simulink model "InverterTestCell2"  (R2021a)
settings: Solver=FixedStepAuto  StartTime=0.0  StopTime=860  FixedStep=0.005  RelTol=1e-3
values from neighbouring files (symbols this model uses):
  ACderate = 0.7910    (= 0.791)    [simvar.m]
  CoreDm = 0.07    [simvar.m]
  CoreRm = 0.250/2    (= 0.125)    [simvar.m]
  Di = 0.085    [Optomised_simvar.m]    (also in simvar.m)
  Dm = 0.08    [simvar.m]
  Hi = 0.250    (= 0.25)    [Optomised_simvar.m]    (also in simvar.m)
  La = 1    [Optomised_simvar.m]    (also in simvar.m = 1.5)
  Li = 0.488    [Optomised_simvar.m]    (also in simvar.m)
  Lw = 1    [Optomised_simvar.m]    (also in simvar.m = 1.5)
  PDi = 0.03    [Optomised_simvar.m]    (also in simvar.m = 0.01)
  PDm = 0.01    [simvar.m]
  PLi = 1    [Optomised_simvar.m]    (also in simvar.m = 3.2)
  PLm = 0.721    [simvar.m]
  PSplit = 0.95    [simvar.m]
  Rm = 0.268/2    (= 0.134)    [simvar.m]
  StartTempI = 295    [simvar.m]
  StartTempM = 291    [simvar.m]
libraries: fl_lib x45, nesl_utility x17
settings Model: PacingRate=0.001800  Creator=Henry  LastModifiedBy=Henry

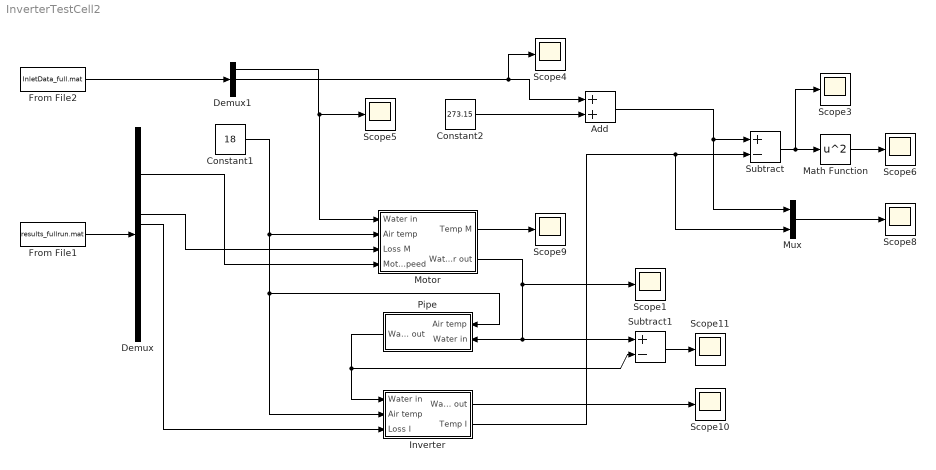
== system InverterTestCell2 ==
  Add : Sum
  Constant1 : Constant  Value=18
  Constant2 : Constant  Value=273.15
  Demux : Demux  Outputs=19
  Demux1 : Demux  Outputs=3
  From File1 : FromFile  FileName=results_fullrun.mat  SampleTime=0
  From File2 : FromFile  FileName=InletData_full.mat  SampleTime=0
  Inverter : Subsystem
  Math Function : Math  Operator=square  SaturateOnIntegerOverflow=on
  Motor : Subsystem
  Mux : Mux  Inputs=2
  Pipe : Subsystem
  Scope{1,3..6,8..11} (9 alike) : Scope
  Subtract : Sum  Inputs=+-
  Subtract1 : Sum  Inputs=+-
  wires:
  From File1/1 -> Demux/1
  Inverter/2(Temp I) -> Mux/2, Subtract/2
  Constant1/1 -> Motor/2(Air temp), Inverter/2(Air temp), Pipe/1(Air temp)
  From File2/1 -> Demux1/1
  Add/1 -> Subtract/1, Mux/1
  Constant2/1 -> Add/2
  Subtract/1 -> Math Function/1, Scope3/1
  Math Function/1 -> Scope6/1
  Mux/1 -> Scope8/1
  Motor/2(Water out) -> Subtract1/1, Pipe/2(Water in), Scope1/1
  Demux/9 -> Inverter/3(Loss I)
  Demux1/1 -> Motor/1(Water in), Scope5/1
  Demux1/2 -> Add/1, Scope4/1
  Demux/4 -> Motor/4(MotorSpeed)
  Demux/8 -> Motor/3(Loss M)
  Motor/1(Temp M) -> Scope9/1
  Inverter/1(Water out) -> Scope10/1
  Pipe/1(Water out) -> Inverter/1(Water in), Subtract1/2
  Subtract1/1 -> Scope11/1

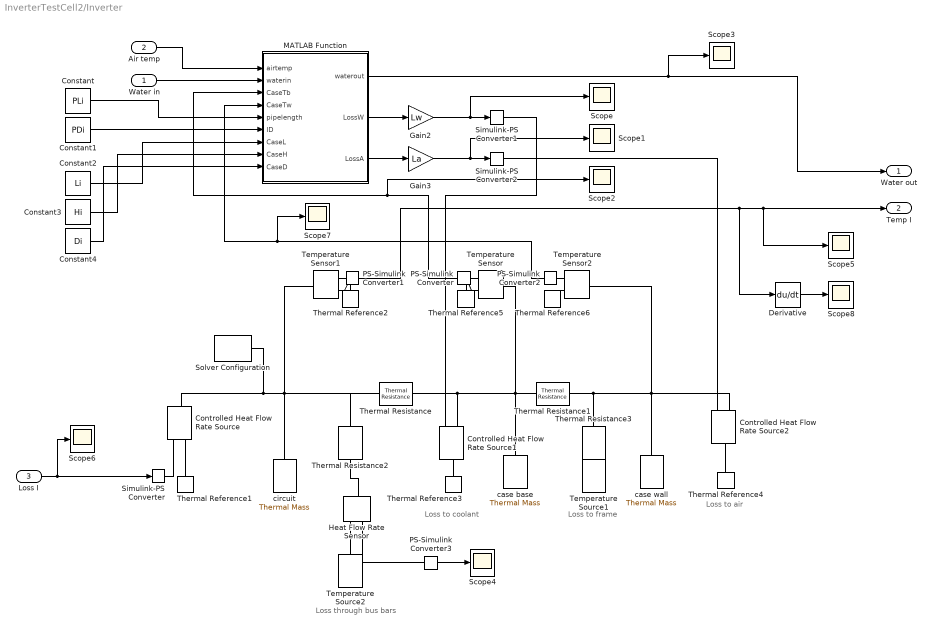
== system InverterTestCell2/Inverter ==
  note: Loss to coolant
  note: Loss to air
  note: Loss through bus
      | bars
  note: Loss to frame
  Water in : Inport
  Air temp : Inport  Port=2
  Loss I : Inport  Port=3
  " case base" : fl_lib/Thermal/Thermal Elements/Thermal Mass  mass=MIbf kg  sp_heat=CpIb J/kg/K  T_specify=on  T_priority=High  T=StartTempI K  T_nominal_specify=off  T_nominal_unit=K  T_nominal_value=1  Q_specify=off  Q_priority=None  Q=0 W  Q_nominal_specify=off  Q_nominal_unit=W  Q_nominal_value=1
  " case wall" : fl_lib/Thermal/Thermal Elements/Thermal Mass  mass=MIbw kg  sp_heat=CpIb J/kg/K  T_specify=on  T_priority=High  T=StartTempI K  T_nominal_specify=off  T_nominal_unit=K  T_nominal_value=1  Q_specify=off  Q_priority=None  Q=0 W  Q_nominal_specify=off  Q_nominal_unit=W  Q_nominal_value=1
  Constant : Constant  Value=PLi
  Constant1 : Constant  Value=PDi
  Constant2 : Constant  Value=Li
  Constant3 : Constant  Value=Hi
  Constant4 : Constant  Value=Di
  Controlled Heat Flow Rate Source : fl_lib/Thermal/Thermal Sources/Controlled Heat Flow Rate Source
  Controlled Heat Flow Rate Source1 : fl_lib/Thermal/Thermal Sources/Controlled Heat Flow Rate Source
  Controlled Heat Flow Rate Source2 : fl_lib/Thermal/Thermal Sources/Controlled Heat Flow Rate Source
  Derivative : Derivative
  Gain2 : Gain  Gain=Lw
  Gain3 : Gain  Gain=La
  Heat Flow Rate Sensor : fl_lib/Thermal/Thermal Sensors/Heat Flow Rate Sensor
      settings: SourceProductBaseCode=SS
  MATLAB Function : MATLAB Function  TreatAsAtomicUnit=on
  PS-Simulink Converter{,1..3} (4 alike) : nesl_utility/PS-Simulink Converter  PhysicalDomain=network_engine_domain  SubClassName=ps_output  LeftPortType=input  RightPortType=output  PseudoPeriodic=off  Frequencies=[]  Unit=inherit  AffineConversion=off
      settings: SourceProductBaseCode=PW,SS
  Scope{,1..8} (9 alike) : Scope
  Simulink-PS Converter : nesl_utility/Simulink-PS Converter  PhysicalDomain=network_engine_domain  SubClassName=ps_input  LeftPortType=input  RightPortType=output  PseudoPeriodic=off  Frequencies=[]  NoiseDistribution=none  NoiseParameters=[]  Unit=1  AffineConversion=off  FilteringAndDerivatives=provide  SimscapeFilterOrder=1  InputFilterTimeConstant=0.001  UdotUserProvided=0
      settings: SourceProductBaseCode=PW,SS
  Simulink-PS Converter1 : nesl_utility/Simulink-PS Converter  PhysicalDomain=network_engine_domain  SubClassName=ps_input  LeftPortType=input  RightPortType=output  PseudoPeriodic=off  Frequencies=[]  NoiseDistribution=none  NoiseParameters=[]  Unit=1  AffineConversion=off  FilteringAndDerivatives=provide  SimscapeFilterOrder=1  InputFilterTimeConstant=0.001  UdotUserProvided=0
      settings: SourceProductBaseCode=PW,SS
  Simulink-PS Converter2 : nesl_utility/Simulink-PS Converter  PhysicalDomain=network_engine_domain  SubClassName=ps_input  LeftPortType=input  RightPortType=output  PseudoPeriodic=off  Frequencies=[]  NoiseDistribution=none  NoiseParameters=[]  Unit=1  AffineConversion=off  FilteringAndDerivatives=provide  SimscapeFilterOrder=1  InputFilterTimeConstant=0.001  UdotUserProvided=0
      settings: SourceProductBaseCode=PW,SS
  Solver Configuration : nesl_utility/Solver Configuration  PhysicalDomain=network_engine_domain  SubClassName=solver  LeftPortType=input  RightPortType=generic  Tones=[]  Harmonics=[]  SimulateNoise=off  Profile=off  UseLocalSampling=off  EnableSwitchedLinearOptims=on  FrequencyDomain=off  UseCCode=off  RelTol=0.001  AbsTol=1e-06  MinStep=1e-09  ToWorkspace=off  RevertToSquareIcSolve=off  NumHomotopyIterations=100  PhasorMode=off  PhasorModeNumHarmonics=1  DoDC=off  ResidualTolerance=1e-09  UseLocalSolver=off  LocalSolverChoice=NE_BACKWARD_EULER_ADVANCER  LocalSolverSampleTime=0.001  DoFixedCost=off  MaxNonlinIter=3  MaxModeIter=2  ComputeImpulses=off  ImpulseIterations=2  LinearAlgebra=auto  EquationFormulation=NE_TIME_EF  DelaysMemoryBudget=2048  AutomaticFiltering=on  FilteringTimeConstant=0.001  PartitionStorageMethod=AS_NEEDED  PartitionMemoryBudget=1024  PartitionMethod=ROBUST
      settings: SourceProductBaseCode=PW,SS
  Temperature Sensor : fl_lib/Thermal/Thermal Sensors/Temperature Sensor
  Temperature Sensor1 : fl_lib/Thermal/Thermal Sensors/Temperature Sensor
  Temperature Sensor2 : fl_lib/Thermal/Thermal Sensors/Temperature Sensor
  Temperature Source1 : fl_lib/Thermal/Thermal Sources/Temperature Source  temperature=293.15 K
  Temperature Source2 : fl_lib/Thermal/Thermal Sources/Temperature Source  temperature=293.15 K
  Thermal Reference{1..6} (6 alike) : fl_lib/Thermal/Thermal Elements/Thermal Reference
  Thermal Resistance : fl_lib/Thermal/Thermal Elements/Thermal Resistance  resistance=Rcb K/W  T_specify=off  T_priority=None  T=0 K  T_nominal_specify=off  T_nominal_unit=K  T_nominal_value=1  Q_specify=off  Q_priority=None  Q=0 W  Q_nominal_specify=off  Q_nominal_unit=W  Q_nominal_value=1
      settings: SourceProductBaseCode=SS
  Thermal Resistance1 : fl_lib/Thermal/Thermal Elements/Thermal Resistance  resistance=Rba K/W  T_specify=off  T_priority=None  T=0 K  T_nominal_specify=off  T_nominal_unit=K  T_nominal_value=1  Q_specify=off  Q_priority=None  Q=0 W  Q_nominal_specify=off  Q_nominal_unit=W  Q_nominal_value=1
      settings: SourceProductBaseCode=SS
  Thermal Resistance2 : fl_lib/Thermal/Thermal Elements/Thermal Resistance  resistance=Rcbb K/W  T_specify=off  T_priority=None  T=0 K  T_nominal_specify=off  T_nominal_unit=K  T_nominal_value=1  Q_specify=off  Q_priority=None  Q=0 W  Q_nominal_specify=off  Q_nominal_unit=W  Q_nominal_value=1
      settings: SourceProductBaseCode=SS
  Thermal Resistance3 : fl_lib/Thermal/Thermal Elements/Thermal Resistance  resistance=Rcf K/W  T_specify=off  T_priority=None  T=0 K  T_nominal_specify=off  T_nominal_unit=K  T_nominal_value=1  Q_specify=off  Q_priority=None  Q=0 W  Q_nominal_specify=off  Q_nominal_unit=W  Q_nominal_value=1
      settings: SourceProductBaseCode=SS
  circuit : fl_lib/Thermal/Thermal Elements/Thermal Mass  mass=MIc kg  sp_heat=CpIc J/kg/K  T_specify=on  T_priority=High  T=StartTempI K  T_nominal_specify=off  T_nominal_unit=K  T_nominal_value=1  Q_specify=off  Q_priority=None  Q=0 W  Q_nominal_specify=off  Q_nominal_unit=W  Q_nominal_value=1
  Water out : Outport  VectorParamsAs1DForOutWhenUnconnected=off
  Temp I : Outport  Port=2  VectorParamsAs1DForOutWhenUnconnected=off
  wires:
  PS-Simulink Converter1/1 -> Temp I/1, Scope5/1, Derivative/1
  Air temp/1 -> MATLAB Function/1(airtemp)
  Water in/1 -> MATLAB Function/2(waterin)
  MATLAB Function/1(waterout) -> Scope3/1, Water out/1
  PS-Simulink Converter/1 -> Scope2/1, MATLAB Function/3(CaseTb)
  MATLAB Function/2(LossW) -> Gain2/1
  MATLAB Function/3(LossA) -> Gain3/1
  Constant/1 -> MATLAB Function/5(pipelength)
  Constant1/1 -> MATLAB Function/6(ID)
  Constant2/1 -> MATLAB Function/7(CaseL)
  Constant3/1 -> MATLAB Function/8(CaseH)
  Constant4/1 -> MATLAB Function/9(CaseD)
  PS-Simulink Converter2/1 -> Scope7/1, MATLAB Function/4(CaseTw)
  Derivative/1 -> Scope8/1
  Loss I/1 -> Simulink-PS Converter/1, Scope6/1
  Gain2/1 -> Scope/1, Simulink-PS Converter1/1
  Gain3/1 -> Scope1/1, Simulink-PS Converter2/1
  PS-Simulink Converter3/1 -> Scope4/1
  connections:
  Thermal Reference3/LConn1 -- Controlled Heat Flow Rate Source1/LConn1
  Thermal Resistance/RConn1 -- Temperature Sensor/LConn1 -- Thermal Resistance1/LConn1 -- " case base"/LConn1 -- Controlled Heat Flow Rate Source1/RConn2
  PS-Simulink Converter/LConn1 -- Temperature Sensor/RConn2
  Controlled Heat Flow Rate Source/RConn2 -- Thermal Reference1/LConn1
  Controlled Heat Flow Rate Source/RConn1 -- Simulink-PS Converter/RConn1
  Thermal Resistance1/RConn1 -- Thermal Resistance3/LConn1 -- Temperature Sensor2/LConn1 -- " case wall"/LConn1 -- Controlled Heat Flow Rate Source2/RConn2
  PS-Simulink Converter1/LConn1 -- Temperature Sensor1/RConn2
  Simulink-PS Converter1/RConn1 -- Controlled Heat Flow Rate Source1/RConn1
  Simulink-PS Converter2/RConn1 -- Controlled Heat Flow Rate Source2/RConn1
  Thermal Reference4/LConn1 -- Controlled Heat Flow Rate Source2/LConn1
  Thermal Reference2/LConn1 -- Temperature Sensor1/RConn1
  Thermal Reference5/LConn1 -- Temperature Sensor/RConn1
  Controlled Heat Flow Rate Source/LConn1 -- Thermal Resistance2/LConn1 -- Thermal Resistance/LConn1 -- Temperature Sensor1/LConn1 -- circuit/LConn1 -- Solver Configuration/RConn1
  PS-Simulink Converter2/LConn1 -- Temperature Sensor2/RConn2
  Temperature Sensor2/RConn1 -- Thermal Reference6/LConn1
  Temperature Source1/LConn1 -- Thermal Resistance3/RConn1
  Heat Flow Rate Sensor/LConn1 -- Thermal Resistance2/RConn1
  Heat Flow Rate Sensor/RConn2 -- Temperature Source2/LConn1
  PS-Simulink Converter3/LConn1 -- Heat Flow Rate Sensor/RConn1

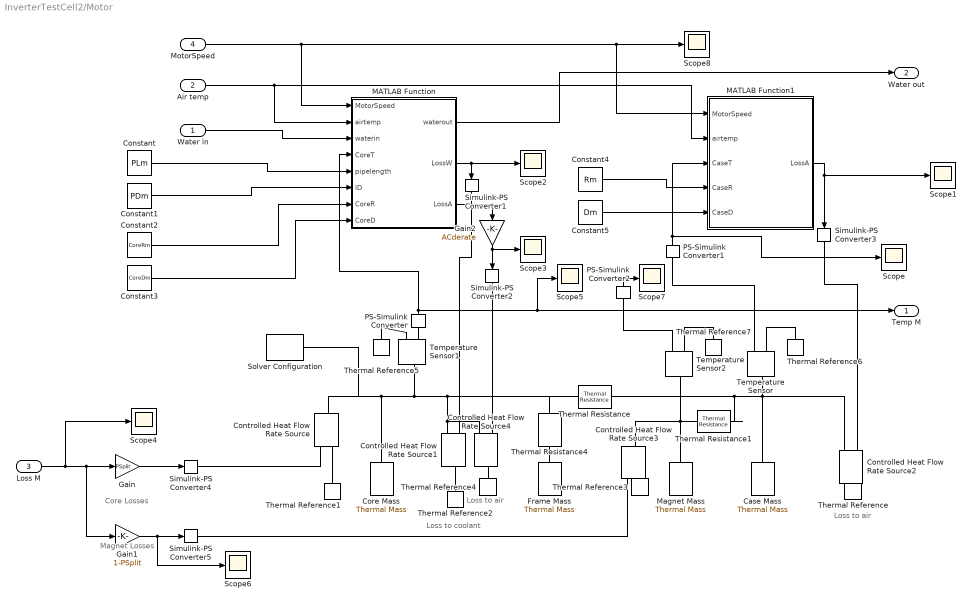
== system InverterTestCell2/Motor ==
  note: Core Losses
  note: Loss to air
  note: Loss to coolant
  note: Loss to air
  note: Magnet Losses
  Water in : Inport
  Air temp : Inport  Port=2
  Loss M : Inport  Port=3
  MotorSpeed : Inport  Port=4
  " Case Mass" : fl_lib/Thermal/Thermal Elements/Thermal Mass  mass=Mcase kg  sp_heat=Cpcase J/kg/K  T_specify=on  T_priority=High  T=StartTempM K  T_nominal_specify=off  T_nominal_unit=K  T_nominal_value=1  Q_specify=off  Q_priority=None  Q=0 W  Q_nominal_specify=off  Q_nominal_unit=W  Q_nominal_value=1
  " Frame Mass" : fl_lib/Thermal/Thermal Elements/Thermal Mass  mass=30 kg  sp_heat=447 J/kg/K  T_specify=on  T_priority=High  T=StartTempM K  T_nominal_specify=off  T_nominal_unit=K  T_nominal_value=1  Q_specify=off  Q_priority=None  Q=0 W  Q_nominal_specify=off  Q_nominal_unit=W  Q_nominal_value=1
  " Magnet Mass" : fl_lib/Thermal/Thermal Elements/Thermal Mass  mass=Mmag kg  sp_heat=Cpmag J/kg/K  T_specify=on  T_priority=High  T=StartTempM K  T_nominal_specify=off  T_nominal_unit=K  T_nominal_value=1  Q_specify=off  Q_priority=None  Q=0 W  Q_nominal_specify=off  Q_nominal_unit=W  Q_nominal_value=1
  Constant : Constant  Value=PLm
  Constant1 : Constant  Value=PDm
  Constant2 : Constant  Value=CoreRm
  Constant3 : Constant  Value=CoreDm
  Constant4 : Constant  Value=Rm
  Constant5 : Constant  Value=Dm
  Controlled Heat Flow Rate Source{,1..4} (5 alike) : fl_lib/Thermal/Thermal Sources/Controlled Heat Flow Rate Source
  Core Mass : fl_lib/Thermal/Thermal Elements/Thermal Mass  mass=Mc kg  sp_heat=Cpcore J/kg/K  T_specify=on  T_priority=High  T=StartTempM K  T_nominal_specify=off  T_nominal_unit=K  T_nominal_value=1  Q_specify=off  Q_priority=None  Q=0 W  Q_nominal_specify=off  Q_nominal_unit=W  Q_nominal_value=1
  Gain : Gain  Gain=PSplit
  Gain1 : Gain  Gain=1-PSplit
  Gain2 : Gain  Gain=ACderate
  MATLAB Function : MATLAB Function  TreatAsAtomicUnit=on
  MATLAB Function1 : MATLAB Function  TreatAsAtomicUnit=on
  PS-Simulink Converter : nesl_utility/PS-Simulink Converter  PhysicalDomain=network_engine_domain  SubClassName=ps_output  LeftPortType=input  RightPortType=output  PseudoPeriodic=off  Frequencies=[]  Unit=inherit  AffineConversion=off
      settings: SourceProductBaseCode=PW,SS
  PS-Simulink Converter1 : nesl_utility/PS-Simulink Converter  PhysicalDomain=network_engine_domain  SubClassName=ps_output  LeftPortType=input  RightPortType=output  PseudoPeriodic=off  Frequencies=[]  Unit=inherit  AffineConversion=off
      settings: SourceProductBaseCode=PW,SS
  PS-Simulink Converter2 : nesl_utility/PS-Simulink Converter  PhysicalDomain=network_engine_domain  SubClassName=ps_output  LeftPortType=input  RightPortType=output  PseudoPeriodic=off  Frequencies=[]  Unit=inherit  AffineConversion=off
      settings: SourceProductBaseCode=PW,SS
  Scope{,1..8} (9 alike) : Scope
  Simulink-PS Converter{1..5} (5 alike) : nesl_utility/Simulink-PS Converter  PhysicalDomain=network_engine_domain  SubClassName=ps_input  LeftPortType=input  RightPortType=output  PseudoPeriodic=off  Frequencies=[]  NoiseDistribution=none  NoiseParameters=[]  Unit=1  AffineConversion=off  FilteringAndDerivatives=provide  SimscapeFilterOrder=1  InputFilterTimeConstant=0.001  UdotUserProvided=0
      settings: SourceProductBaseCode=PW,SS
  Solver Configuration : nesl_utility/Solver Configuration  PhysicalDomain=network_engine_domain  SubClassName=solver  LeftPortType=input  RightPortType=generic  Tones=[]  Harmonics=[]  SimulateNoise=off  Profile=off  UseLocalSampling=off  EnableSwitchedLinearOptims=on  FrequencyDomain=off  UseCCode=off  RelTol=0.001  AbsTol=1e-06  MinStep=1e-09  ToWorkspace=off  RevertToSquareIcSolve=off  NumHomotopyIterations=100  PhasorMode=off  PhasorModeNumHarmonics=1  DoDC=off  ResidualTolerance=1e-09  UseLocalSolver=off  LocalSolverChoice=NE_BACKWARD_EULER_ADVANCER  LocalSolverSampleTime=0.001  DoFixedCost=off  MaxNonlinIter=3  MaxModeIter=2  ComputeImpulses=off  ImpulseIterations=2  LinearAlgebra=auto  EquationFormulation=NE_TIME_EF  DelaysMemoryBudget=2048  AutomaticFiltering=on  FilteringTimeConstant=0.001  PartitionStorageMethod=AS_NEEDED  PartitionMemoryBudget=1024  PartitionMethod=ROBUST
      settings: SourceProductBaseCode=PW,SS
  Temperature Sensor : fl_lib/Thermal/Thermal Sensors/Temperature Sensor
  Temperature Sensor1 : fl_lib/Thermal/Thermal Sensors/Temperature Sensor
  Temperature Sensor2 : fl_lib/Thermal/Thermal Sensors/Temperature Sensor
  Thermal Reference{,1..7} (8 alike) : fl_lib/Thermal/Thermal Elements/Thermal Reference
  Thermal Resistance : fl_lib/Thermal/Thermal Elements/Thermal Resistance  resistance=Rcc K/W  T_specify=off  T_priority=None  T=0 K  T_nominal_specify=off  T_nominal_unit=K  T_nominal_value=1  Q_specify=off  Q_priority=None  Q=0 W  Q_nominal_specify=off  Q_nominal_unit=W  Q_nominal_value=1
      settings: SourceProductBaseCode=SS
  Thermal Resistance1 : fl_lib/Thermal/Thermal Elements/Thermal Resistance  resistance=Rmc K/W  T_specify=off  T_priority=None  T=0 K  T_nominal_specify=off  T_nominal_unit=K  T_nominal_value=1  Q_specify=off  Q_priority=None  Q=0 W  Q_nominal_specify=off  Q_nominal_unit=W  Q_nominal_value=1
      settings: SourceProductBaseCode=SS
  Thermal Resistance4 : fl_lib/Thermal/Thermal Elements/Thermal Resistance  resistance=Rcf K/W  T_specify=off  T_priority=None  T=0 K  T_nominal_specify=off  T_nominal_unit=K  T_nominal_value=1  Q_specify=off  Q_priority=None  Q=0 W  Q_nominal_specify=off  Q_nominal_unit=W  Q_nominal_value=1
      settings: SourceProductBaseCode=SS
  Temp M : Outport  VectorParamsAs1DForOutWhenUnconnected=off
  Water out : Outport  Port=2  VectorParamsAs1DForOutWhenUnconnected=off
  wires:
  PS-Simulink Converter/1 -> Scope5/1, Temp M/1, MATLAB Function/4(CoreT)
  Air temp/1 -> MATLAB Function1/2(airtemp), MATLAB Function/2(airtemp)
  Water in/1 -> MATLAB Function/3(waterin)
  MATLAB Function/2(LossW) -> Scope2/1, Simulink-PS Converter1/1
  MATLAB Function/3(LossA) -> Gain2/1
  MATLAB Function/1(waterout) -> Water out/1
  MATLAB Function1/1(LossA) -> Scope1/1, Simulink-PS Converter3/1
  PS-Simulink Converter1/1 -> MATLAB Function1/3(CaseT), Scope/1
  Loss M/1 -> Scope4/1, Gain/1, Gain1/1
  Gain/1 -> Simulink-PS Converter4/1
  Gain1/1 -> Scope6/1, Simulink-PS Converter5/1
  Constant/1 -> MATLAB Function/5(pipelength)
  Constant1/1 -> MATLAB Function/6(ID)
  Constant2/1 -> MATLAB Function/7(CoreR)
  Constant3/1 -> MATLAB Function/8(CoreD)
  Constant4/1 -> MATLAB Function1/4(CaseR)
  Constant5/1 -> MATLAB Function1/5(CaseD)
  MotorSpeed/1 -> MATLAB Function/1(MotorSpeed), MATLAB Function1/1(MotorSpeed), Scope8/1
  PS-Simulink Converter2/1 -> Scope7/1
  Gain2/1 -> Scope3/1, Simulink-PS Converter2/1
  connections:
  Thermal Resistance/RConn1 -- Thermal Resistance1/RConn1 -- Temperature Sensor/LConn1 -- " Case Mass"/LConn1 -- Controlled Heat Flow Rate Source2/RConn2
  Simulink-PS Converter4/RConn1 -- Controlled Heat Flow Rate Source/RConn1
  Thermal Reference/LConn1 -- Controlled Heat Flow Rate Source2/LConn1
  Controlled Heat Flow Rate Source/RConn2 -- Thermal Reference1/LConn1
  PS-Simulink Converter/LConn1 -- Temperature Sensor1/RConn2
  Controlled Heat Flow Rate Source1/LConn1 -- Thermal Reference2/LConn1
  Thermal Reference3/LConn1 -- Controlled Heat Flow Rate Source3/RConn2
  Thermal Reference4/LConn1 -- Controlled Heat Flow Rate Source4/LConn1
  Simulink-PS Converter1/RConn1 -- Controlled Heat Flow Rate Source1/RConn1
  Simulink-PS Converter2/RConn1 -- Controlled Heat Flow Rate Source4/RConn1
  Simulink-PS Converter3/RConn1 -- Controlled Heat Flow Rate Source2/RConn1
  PS-Simulink Converter1/LConn1 -- Temperature Sensor/RConn2
  Simulink-PS Converter5/RConn1 -- Controlled Heat Flow Rate Source3/RConn1
  Controlled Heat Flow Rate Source4/RConn2 -- Controlled Heat Flow Rate Source1/RConn2 -- Solver Configuration/RConn1 -- Controlled Heat Flow Rate Source/LConn1 -- Core Mass/LConn1 -- Temperature Sensor1/LConn1 -- Thermal Resistance/LConn1 -- Thermal Resistance4/LConn1
  Thermal Resistance4/RConn1 -- " Frame Mass"/LConn1
  Thermal Reference5/LConn1 -- Temperature Sensor1/RConn1
  Temperature Sensor/RConn1 -- Thermal Reference6/LConn1
  Controlled Heat Flow Rate Source3/LConn1 -- Temperature Sensor2/LConn1 -- Thermal Resistance1/LConn1 -- " Magnet Mass"/LConn1
  Temperature Sensor2/RConn1 -- Thermal Reference7/LConn1
  PS-Simulink Converter2/LConn1 -- Temperature Sensor2/RConn2

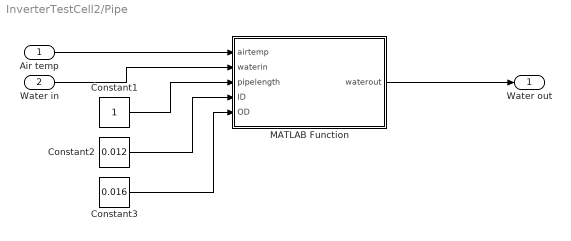
== system InverterTestCell2/Pipe ==
  Air temp : Inport
  Water in : Inport  Port=2
  Constant1 : Constant
  Constant2 : Constant  Value=0.012
  Constant3 : Constant  Value=0.016
  MATLAB Function : MATLAB Function  TreatAsAtomicUnit=on
  Water out : Outport  VectorParamsAs1DForOutWhenUnconnected=off
  wires:
  MATLAB Function/1(waterout) -> Water out/1
  Constant1/1 -> MATLAB Function/3(pipelength)
  Water in/1 -> MATLAB Function/2(waterin)
  Air temp/1 -> MATLAB Function/1(airtemp)
  Constant2/1 -> MATLAB Function/4(ID)
  Constant3/1 -> MATLAB Function/5(OD)

== matlab function InverterTestCell2/Pipe/MATLAB Function ==
  data: airtemp input; waterin input; waterout output; pipelength input; ID input; OD input
function waterout = Pipefcn(airtemp,waterin,pipelength,ID,OD)

L = pipelength;
AveWtemp = waterin;
kpipe = 0.13;
dm = 0.1;
u = (dm/1000)/(pi()*((ID/2)^2));
filmT1 = (waterin + airtemp)/2;
filmT2 = (waterin + airtemp)/2;

for x = 1:3
    [Rew,Prw,Grw,kw,Cpw] = Variablefinder('water',filmT1,AveWtemp,u,ID);
    [Rea,Pra,Gra,ka,Cpa] = Variablefinder('air',filmT2,airtemp,0,OD);
    
    if Rew <= 2300
        Nuw = 3.66;     %value for laminar flow in a pipe with constant surface temp
    else
       Nuw = 0.023*(Rew^(4/5))*(Prw^0.3);   %equation for turbulent flow in a cooling pipe
    end
    
    Raa = Pra*Gra;  %calculate the rayleigh number
    HorNua = (0.6 + ( (0.387*(Raa^(1/6))) / ((1 + ((0.559/Pra)^(9/16)))^(8/27)) ) )^2;
    VertNua = (0.825 + ( (0.387*(Raa^(1/6))) / ((1 + ((0.492/Pra)^(9/16)))^(8/27)) ) )^2;
    Nua = 1*HorNua + 0*VertNua;
    
    h1 = Nuw*kw/ID;
    h2 = Nua*ka/OD;

    R1 = 1/(2*pi()*(ID/2)*L*h1);
    R2 = (log((OD/2)/(ID/2)))/(2*pi()*L*kpipe);
    R3 = 1/(2*pi()*(OD/2)*L*h2);
    Rt = R1 + R2 + R3;
    
    waterout = airtemp - (airtemp-waterin)*exp(-1/(dm*Cpw*Rt));

    AveWtemp = (waterin + waterout)/2;
    AvedQ = dm*Cpw*(waterin - waterout);
    
    dT1 = AvedQ*R1;
    %dT2 = AvedQ*R2;
    dT3 = AvedQ*R3;
    
    filmT1 = AveWtemp + (dT1/2);
    filmT2 = airtemp - (dT3/2);   
end

end

== matlab function InverterTestCell2/Inverter/MATLAB Function ==
  data: airtemp input; waterin input; CaseTb input; CaseTw input; waterout output; pipelength input; ID input; CaseL input; CaseH input; CaseD input; LossW output; LossA output
function [waterout,LossW,LossA] = Invfcn(airtemp,waterin,CaseTb,CaseTw,pipelength,ID,CaseL,CaseH,CaseD)

CaseTb = CaseTb - 273.15;
CaseTw = CaseTw - 273.15;
u = (0.0001)/(pi()*((ID/2)^2));
dmw = 0.0001*1000;
L = pipelength;
AveWtemp = waterin;
filmT1 = (waterin + CaseTb)/2;
filmT2 = (CaseTw + airtemp)/2;

[Rew,Prw,Grw,kw,Cpw] = Variablefinder('water',filmT1,AveWtemp,u,ID);
[Rea,Pra,Gra,ka,Cpa] = Variablefinder('air',filmT2,airtemp,0,CaseH);

if Rew <= 2300
    Nuw = 3.66;     %value for laminar flow in a pipe with constant surface temp
else
    Nuw = 0.023*(Rew^(4/5))*(Prw^0.3);   %equation for turbulent flow in a cooling pipe
end

Raa = Pra*Gra;  %calculate the rayleigh number
Nua = (0.825 + ( (0.387*(Raa^(1/6))) / ((1 + ((0.492/Pra)^(9/16)))^(8/27)) ) )^2;

h1 = Nuw*kw/(ID);
h2 = Nua*ka/CaseH;

R1 = 1/(2*pi()*(ID/2)*L*h1);

R2 = 1/(((2*CaseL*CaseH)+(2*CaseH*CaseD))*h2);

waterout = CaseTb - (CaseTb-waterin)*exp(-1/(dmw*Cpw*R1));

LossW = dmw*Cpw*(waterout - waterin);

LossA = (CaseTw-airtemp)/R2;

end

== matlab function InverterTestCell2/Motor/MATLAB Function ==
  data: MotorSpeed input; airtemp input; waterin input; CoreT input; waterout output; pipelength input; ID input; CoreR input; CoreD input; LossW output; LossA output
function [waterout,LossW,LossA] = MotCorefcn(MotorSpeed,airtemp,waterin,CoreT,pipelength,ID,CoreR,CoreD)

SurfSpeed = (abs(MotorSpeed)/CoreR)+0.6;
CoreT = CoreT - 273.15;
L = pipelength;
AveWtemp = waterin;
dmw = 0.1;
u = (dmw/1000)/(pi()*((ID/2)^2));
filmT1 = (waterin + CoreT)/2;
filmT2 = (CoreT + airtemp)/2;

[Rew,Prw,Grw,kw,Cpw] = Variablefinder('water',filmT1,AveWtemp,u,ID);
[Rea,Pra,Gra,ka,Cpa] = Variablefinder('air',filmT2,airtemp,SurfSpeed,pi()*CoreR*2);

if Rew <= 2300
    Nuw = 3.66;     %value for laminar flow in a pipe with constant surface temp
else
    Nuw = 0.023*(Rew^(4/5))*(Prw^0.3);   %equation for turbulent flow in a cooling pipe
end

% Raa = Pra*Gra;  %calculate the rayleigh number
% Nua = (0.825 + ( (0.387*(Raa^(1/6))) / ((1 + ((0.492/Pra)^(9/16)))^(8/27)) ) )^2;
if Rea <= (5*10^5)
    Nua = 0.664*(Rea^(1/2))*(Pra^(1/3));
else
    Nua = ((0.037*(Rea^(4/5)))-871)*(Pra^(1/3));
end

h1 = Nuw*kw/(ID);
h2 = Nua*ka/pi()*CoreR*2;

R1 = 1/(pi()*(ID)*L*h1);

R2 = 1/((pi()*(CoreD)*2*CoreR*h2));

waterout = CoreT - (CoreT-waterin)*exp(-1/(dmw*Cpw*R1));

LossW = dmw*Cpw*(waterout - waterin);

LossA = (CoreT-airtemp)/R2;

end

== matlab function InverterTestCell2/Motor/MATLAB Function1 ==
  data: MotorSpeed input; airtemp input; CaseT input; CaseR input; CaseD input; LossA output
function LossA  = MotCasefcn(MotorSpeed,airtemp,CaseT,CaseR,CaseD)

SurfSpeed = abs(MotorSpeed)/CaseR;
CaseT = CaseT - 273.15;
filmT1 = (CaseT + airtemp)/2;

[Rea,Pra,Gra,ka,Cpa] = Variablefinder('air',filmT1,airtemp,SurfSpeed,pi()*CaseR*2);

if Rea <= (5*10^5)
    Nua = 0.664*(Rea^(1/2))*(Pra^(1/3));
else
    Nua = ((0.037*(Rea^(4/5)))-871)*(Pra^(1/3));
end

h1 = Nua*ka/(2*CaseR*pi());

R1 = 1/((2*CaseR*pi())*CaseD*h1);

LossA = (CaseT-airtemp)/R1;

end
